simulink model "exampleIAM_b0"  (R2013b)
settings: Solver=ode45  StartTime=0  StopTime=100  RelTol=1e-3
undefined symbols (not defined in the file): Incidence_Angle_sun, Solar_Radiation_diffuse_surface, Solar_Radiation_direct_surface
libraries: simulink x3, carnot x2, simulink_extras x1
settings Model: Creator=drhf  LastModifiedBy=drhf
settings OptimizationCC: ExpressionDepthLimit=2147483647
settings DebuggingCC: StateNameClashWarn=warning
settings GRTTargetCC: CombineOutputUpdateFcns=off  GRTInterface=on

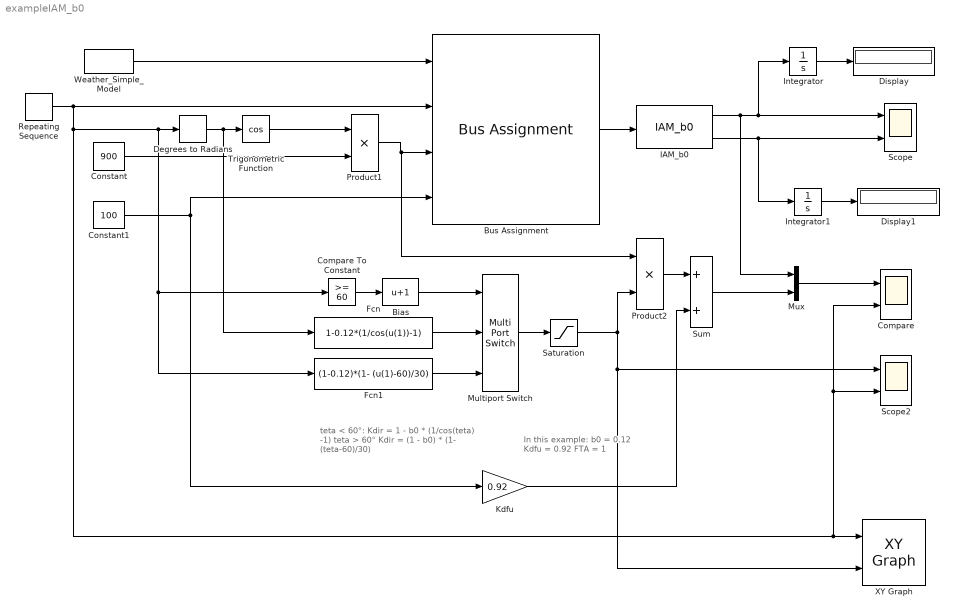
== system exampleIAM_b0 ==
  note: teta < 60°:
      | Kdir = 1 - b0 * (1/cos(teta) -1)
      | teta > 60°
      | Kdir = (1 - b0) * (1- (teta-60)/30)
  note: In this example:
      | b0 = 0.12
      | Kdfu = 0.92
      | FTA = 1
  Bias : Bias  Bias=1
  Bus Assignment : BusAssignment  AssignedSignals=Incidence_Angle_sun,Solar_Radiation_direct_surface,Solar_Radiation_diffuse_surface
  Compare : Scope  NumInputPorts=2
      settings: YMin=-5~-5  YMax=5~5
  Compare To Constant : simulink/Logic and Bit Operations/Compare To Constant  relop=>=  const=60  OutDataTypeStr=uint8
  Constant : Constant  Value=900
  Constant1 : Constant  Value=100
  Degrees to Radians : simulink_extras/Transformations/Degrees to Radians
  Display : Display
  Display1 : Display
  Fcn : Fcn  Expr=1-0.12*(1/cos(u(1))-1)
  Fcn1 : Fcn  Expr=(1-0.12)*(1- (u(1)-60)/30)
  IAM_b0 : carnot/Source/Solar_Thermal/IncidenceAngleModifier/IAM_b0  b0=0.12  Kd=0.92  fta=1
  Integrator : Integrator
  Integrator1 : Integrator
  Kdfu : Gain  Gain=0.92
  Multiport Switch : MultiPortSwitch  Inputs=2
  Mux : Mux  Inputs=2
  Product1 : Product  RndMeth=Zero
  Product2 : Product  RndMeth=Zero
  Repeating Sequence : simulink/Sources/Repeating Sequence  rep_seq_t=[0 90 120]  rep_seq_y=[0 90 90]
  Saturation : Saturate  UpperLimit=inf  LowerLimit=0
  Scope : Scope  NumInputPorts=2
      settings: YMin=-5~-5  YMax=5~5
  Scope2 : Scope  NumInputPorts=2
      settings: YMin=-5~-5  YMax=5~5  SaveName=ScopeData2
  Sum : Sum  SaturateOnIntegerOverflow=on  InputSameDT=on  OutDataTypeStr=Inherit: Same as first input
  Trigonometric Function : Trigonometry  Operator=cos
  Weather_Simple_Model : carnot/Weather/Weather_Simple_Model  lat=60  Ibn=900  Idg=100  tamb=5  deltaTsky=-6  rh=50  precip="10e-3/24/3600           % 10 mm in 24 h"  cloud=0.125  p=1013e2  vw=1  wdir=270
  XY Graph : simulink/Sinks/XY Graph  xmin=0  xmax=90  ymin=0  ymax=1  st=-1
  wires:
  IAM_b0/1 -> Scope/1, Integrator/1, Mux/1
  IAM_b0/2 -> Integrator1/1, Scope/2
  Integrator/1 -> Display/1
  Weather_Simple_Model/1 -> Bus Assignment/1
  Bus Assignment/1 -> IAM_b0/1
  Repeating Sequence/1 -> Bus Assignment/2, Compare To Constant/1, Fcn1/1, Degrees to Radians/1, Compare/2, Scope2/2, XY Graph/1
  Degrees to Radians/1 -> Trigonometric Function/1, Fcn/1
  Trigonometric Function/1 -> Product1/1
  Integrator1/1 -> Display1/1
  Kdfu/1 -> Sum/2
  Product2/1 -> Sum/1
  Fcn/1 -> Multiport Switch/2
  Sum/1 -> Mux/2
  Mux/1 -> Compare/1
  Multiport Switch/1 -> Saturation/1
  Saturation/1 -> Product2/2, XY Graph/2, Scope2/1
  Constant/1 -> Product1/2
  Constant1/1 -> Bus Assignment/4, Kdfu/1
  Fcn1/1 -> Multiport Switch/3
  Compare To Constant/1 -> Bias/1
  Bias/1 -> Multiport Switch/1
  Product1/1 -> Product2/1, Bus Assignment/3
